simulink model "calcul_Mz"  (R2024b)
settings: Solver=FixedStepAuto  StartTime=0.0  StopTime=10.0  FixedStep=Ts  RelTol=1e-3
settings Model: Creator=marti  LastModifiedBy=Filip

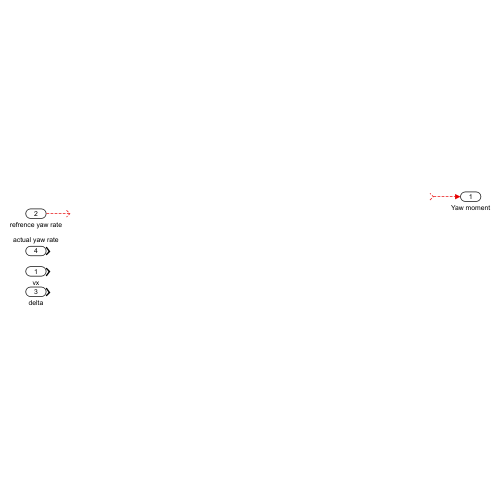
[thumbnail: Simulink's stored preview of the top-level diagram]
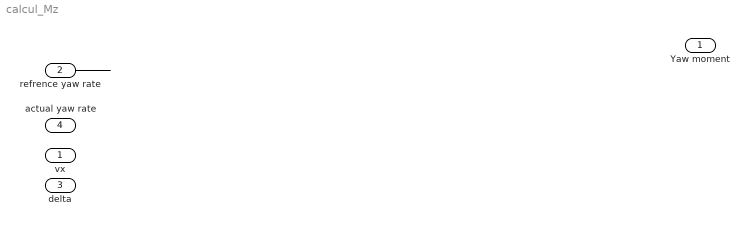
== system calcul_Mz ==
  vx : Inport
  refrence yaw rate : Inport  Port=2
  delta : Inport  Port=3
  actual yaw rate : Inport  Port=4
  Yaw moment : Outport
  wires:
  refrence yaw rate/1 -> ?
  ? -> Yaw moment/1
